simulink subsystem "vector_sin_controller"  (R2023a)
settings: Solver=VariableStepAuto  StartTime=0.0  StopTime=10.0  RelTol=1e-3
settings Model: Creator=motya  LastModifiedBy=motya

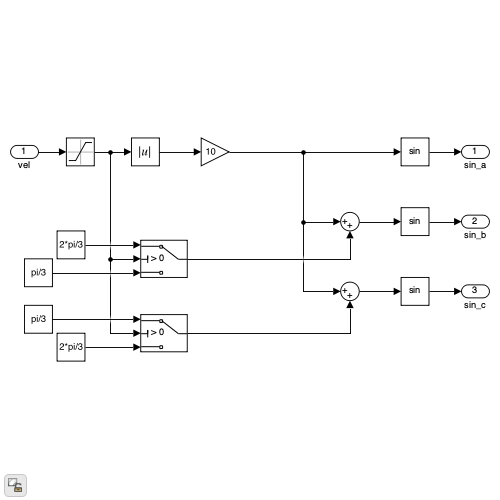
[thumbnail: Simulink's stored preview of the top-level diagram]
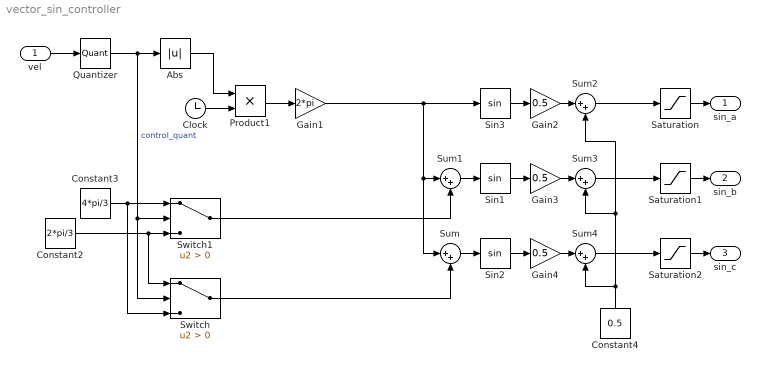
== system vector_sin_controller ==
  vel : Inport
  Abs : Abs  SaturateOnIntegerOverflow=off
  Clock : Clock
  Constant2 : Constant  Value=2*pi/3
  Constant3 : Constant  Value=4*pi/3
  Constant4 : Constant  Value=0.5
  Gain1 : Gain  Gain=2*pi
  Gain2 : Gain  Gain=0.5
  Gain3 : Gain  Gain=0.5
  Gain4 : Gain  Gain=0.5
  Product1 : Product
  Quantizer : Quantizer  QuantizationInterval=2
  Saturation : Saturate  UpperLimit=0.99  LowerLimit=0.001
  Saturation1 : Saturate  UpperLimit=0.99  LowerLimit=0.001
  Saturation2 : Saturate  UpperLimit=0.99  LowerLimit=0.001
  Sin1 : Trigonometry
  Sin2 : Trigonometry
  Sin3 : Trigonometry
  Sum{,1..4} (5 alike) : Sum  Inputs=|++
  Switch : Switch  Criteria=u2 > Threshold  SaturateOnIntegerOverflow=off  InputSameDT=off
  Switch1 : Switch  Criteria=u2 > Threshold  SaturateOnIntegerOverflow=off  InputSameDT=off
  sin_a : Outport
  sin_b : Outport  Port=2
  sin_c : Outport  Port=3
  wires:
  Switch/1 -> Sum/2
  Sum/1 -> Sin2/1
  Sum1/1 -> Sin1/1
  Switch1/1 -> Sum1/2
  Constant3/1 -> Switch1/1, Switch/3
  Constant2/1 -> Switch1/3, Switch/1
  Gain1/1 -> Sum1/1, Sum/1, Sin3/1
  Clock/1 -> Product1/2
  Abs/1 -> Product1/1
  Product1/1 -> Gain1/1
  Sum2/1 -> Saturation/1
  Sum3/1 -> Saturation1/1
  Sum4/1 -> Saturation2/1
  Constant4/1 -> Sum2/2, Sum3/2, Sum4/2
  Sin3/1 -> Gain2/1
  Gain2/1 -> Sum2/1
  Sin1/1 -> Gain3/1
  Gain3/1 -> Sum3/1
  Sin2/1 -> Gain4/1
  Gain4/1 -> Sum4/1
  Saturation/1 -> sin_a/1
  Saturation1/1 -> sin_b/1
  Saturation2/1 -> sin_c/1
  vel/1 -> Quantizer/1
  Quantizer/1 -> Switch/2, Switch1/2, Abs/1  "control_quant"
